simulink model "ModeleControlX"  (R2015a)
settings: Solver=ode3  StartTime=0.0  StopTime=0.2  FixedStep=dt  RelTol=1e-3
values from neighbouring files (symbols this model uses):
  B = 4    [param.m]
  i = 3    [param.m]
  Jeq = I1+Ir+1/i^2*(I3+I6+(m4+m5)*R^2)    (= 0.000214958998807)    [param.m]
  kc = 0.21    [param.m]
  ke = 0.2083    [param.m]
  L = 3.2e-3    (= 0.0032)    [param.m]
  r = 5.1    [param.m]
  R = 155/(2*pi)/1000    (= 0.0246690161792)    [param.m]
settings Model: Creator=Fred  LastModifiedBy=pt_ptsi
settings SolverCC: ZeroCrossControl=EnableAll  ZeroCrossAlgorithm=Adaptive

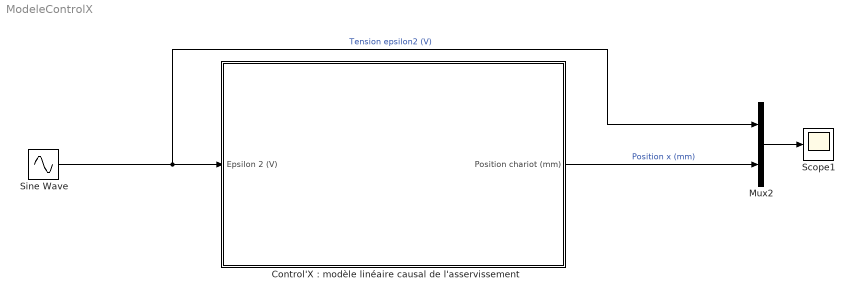
== system ModeleControlX ==
  "Control'X : modèle linéaire causal de l'asservissement" : Subsystem
      mask Display: image('Control''X.jpg')
  Mux2 : Mux  Inputs=2
  Scope1 : Scope
      settings: TimeRange=auto  ShowLegends=on  MaxDataPoints=5000  SaveToWorkspace=off  YMin=-9.99999  YMax=10.00000  SampleTime=-1  DataFormat=Array
  Sine Wave : Sin  Amplitude=8  Frequency=200  SampleTime=0
  wires:
  Sine Wave/1 -> "Control'X : modèle linéaire causal de l'asservissement"/1(Epsilon 2 (V)), Mux2/1  "Tension epsilon2 (V)"
  "Control'X : modèle linéaire causal de l'asservissement"/1(Position chariot (mm)) -> Mux2/2  "Position x (mm)"
  Mux2/1 -> Scope1/1

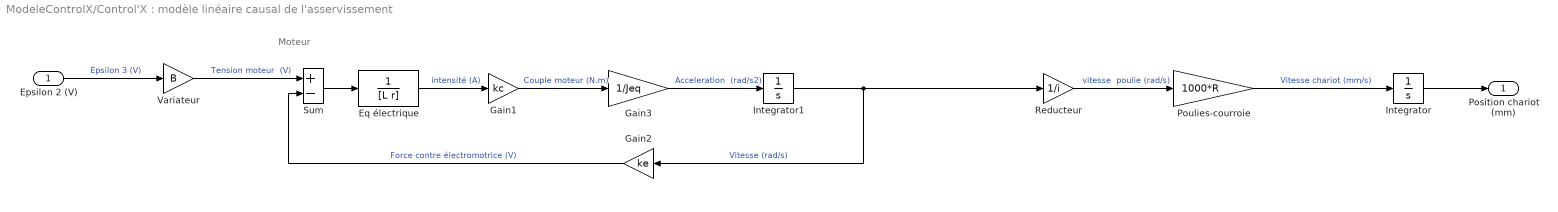
== system ModeleControlX/Control'X : modèle linéaire causal de l'asservissement ==
  note: Moteur
  Epsilon 2 (V) : Inport
  Eq électrique : TransferFcn  Denominator=[L r]
  Gain1 : Gain  Gain=kc
  Gain2 : Gain  Gain=ke
  Gain3 : Gain  Gain=1/Jeq
  Integrator : Integrator
  Integrator1 : Integrator
  Poulies-courroie : Gain  Gain=1000*R
  Reducteur : Gain  Gain=1/i
  Sum : Sum  Inputs=+-
  Variateur : Gain  Gain=B
  Position chariot (mm) : Outport
  wires:
  Eq électrique/1 -> Gain1/1  "intensité (A)"
  Variateur/1 -> Sum/1  "Tension moteur  (V)"
  Integrator1/1 -> Reducteur/1, Gain2/1  "Vitesse (rad/s)"
  Sum/1 -> Eq électrique/1
  Gain2/1 -> Sum/2  "Force contre électromotrice (V)"
  Gain1/1 -> Gain3/1  "Couple moteur (N.m)"
  Poulies-courroie/1 -> Integrator/1  "Vitesse chariot (mm/s)"
  Reducteur/1 -> Poulies-courroie/1  "vitesse  poulie (rad/s)"
  Integrator/1 -> Position chariot (mm)/1
  Gain3/1 -> Integrator1/1  "Acceleration  (rad/s2)"
  Epsilon 2 (V)/1 -> Variateur/1  "Epsilon 3 (V)"
